simulink model "Kundur_BESS_STA_Nov14_2021a_v2_2021a"  (R2023a)
settings: Solver=VariableStepAuto  StartTime=0.0  StopTime=3  FixedStep=Ts  MaxStep=1e-5  MinStep=1e-20  RelTol=1e-3  EnableMultiTasking=on
PreLoadFcn:
  | Ts=50e-6;
PostLoadFcn:
  | Ts=50e-6;
InitFcn:
  | Ts=50e-6;
values from neighbouring files (symbols this model uses):
  current_K_den = [1 -1.95396088137 0.953960881373]    [param_cntrl_v2.mat]
  current_K_num = [292.549944556 -582.765243791 290.215658722]    [param_cntrl_v2.mat]
  flt_den = [1 -1.99914493247 0.999500180349]    [param_cntrl_v2.mat]
  flt_num = [0.000249925443627 3.12366678454e-08 -0.000249894206959]    [param_cntrl_v2.mat]
  flt_rocof_den = [1 -3.94812243331 5.84544117496 -3.84650440967 0.949185710471]    [param_cntrl_v2.mat]
  flt_rocof_num = [2.65341753303e-09 1.06136701321e-08 1.59205051982e-08 1.06136701321e-08 2.65341753303e-09]    [param_cntrl_v2.mat]
  pll_K_den = [1 -1.95396088137 0.953960881373]    [param_cntrl_v2.mat]
  pll_K_num = [1047.77474974 -2078.89023245 1031.12061217]    [param_cntrl_v2.mat]
  sampling_k = 5e-05    [param_cntrl_v2.mat]
undefined symbols (not defined in the file or in its folder): Ad2, Ad4, Bd2, Bd4, Cd2, Cd4, D1, Delta, flt_rocof_a_den, flt_rocof_a_num, flt_rocof_b_den, flt_rocof_b_num, Gd2, Gd4, Kd2, Kd4, L, R
libraries: spsThreePhaseVIMeasurementLib x15, spsLoadFlowBusLib x12, spsSeriesRLCBranchLib x11, spsThreePhaseSeriesRLCLoadLib x11, spsThreePhaseTransformerTwoWindingsLib x8, spsThreePhaseSeriesRLCBranchLib x8, spsabctoAlphaBetaZeroLib x8, spsGenericPowerSystemStabilizerLib x8, spsPowerPositiveSequenceLib x7, spsThreePhaseParallelRLCLoadLib x6, spsPLL3phLib x6, spsGroundLib x6
(part 2 of 4)

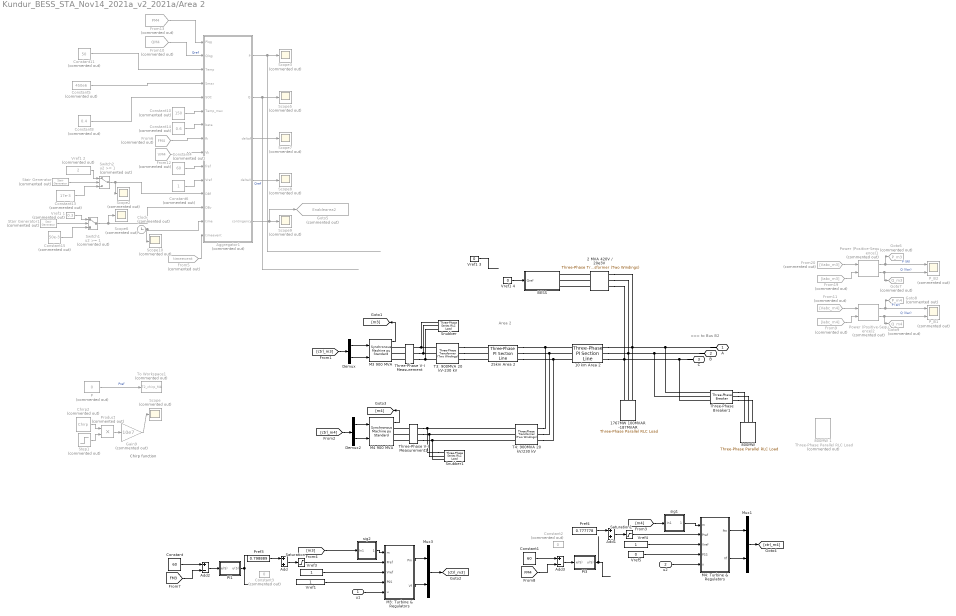
== system Kundur_BESS_STA_Nov14_2021a_v2_2021a/Area 2 ==
  note: ==> to Bus B2
  note: Area 2
  note: Chirp function
  u1 : Inport
  u2 : Inport  Port=2
  10 km Area 2 : spsThreePhasePISectionLineLib/Three-Phase PI Section Line  LConnTagsString=a|b|c  RConnTagsString=A|B|C  Length=10  Frequency=60  Resistances=[0.0001*529 1.61]  Inductances=[0.001*529/(377) 0.0061]  Capacitances=[0.00175/529/(377) 5.2489e-9]
  1767MW 100MVAR -187MVAR : spsThreePhaseParallelRLCLoadLib/Three-Phase Parallel RLC Load  LConnTagsString=A|B|C  Configuration=Y (grounded)  NominalVoltage=230e3  Vabc=[1e3 1e3 1e3]  Vabcp=[1e3 1e3 1e3]  NominalFrequency=60  UnbalancedPower=off  ActivePower=1767e6  InductivePower=0  CapacitivePower=0  Pabc=[10e3 9e3 11e3]  QLabc=[100 90 110]  QCabc=[100 90 110]  Pabcp=[10e3 9e3 11e3]  QLabcp=[100 90 110]  QCabcp=[100 90 110]  Measurements=None  LoadType=constant Z
  2 MVA 420V / 20e3V : spsThreePhaseTransformerTwoWindingsLib/Three-Phase Transformer (Two Windings)  Winding1Connection=Delta (D1)  Winding2Connection=Yg  CoreType=Three single-phase transformers  SetSaturation=off  Hysteresis=off  DataFile='hysteresis'  SetInitialFlux=off  Measurements=None  UNITS=pu  NominalPower=[900e6 , 60 ]  Winding1=[ 20e3 , 0.001 , 0.03 ]  Winding2=[ 420 , 0.001 , 0.03 ]  Rm=500  Lm=500  L0=0.5  Saturation=[ 0,0 ; 0.0024,1.2 ; 1.0,1.52 ]  InitialFluxes=[0.79999 -0.79999 0.7]  BreakLoop=off  DiscreteSolver=Trapezoidal iterative  DataType=off  TransfoNumber=0
  25km Area 2 : spsThreePhasePISectionLineLib/Three-Phase PI Section Line  LConnTagsString=a|b|c  RConnTagsString=A|B|C  Length=25  Frequency=60  Resistances=[0.0001*529 1.61]  Inductances=[0.001*529/(377) 0.0061]  Capacitances=[0.00175/529/(377) 5.2489e-9]
  "800MW " : spsThreePhaseParallelRLCLoadLib/Three-Phase Parallel RLC Load  LConnTagsString=A|B|C  Configuration=Y (grounded)  NominalVoltage=230e3  Vabc=[1e3 1e3 1e3]  Vabcp=[1e3 1e3 1e3]  NominalFrequency=60  UnbalancedPower=off  ActivePower=150e6  InductivePower=0  CapacitivePower=0  Pabc=[10e3 9e3 11e3]  QLabc=[100 90 110]  QCabc=[100 90 110]  Pabcp=[10e3 9e3 11e3]  QLabcp=[100 90 110]  QCabcp=[100 90 110]  Measurements=None  LoadType=constant Z
  800MW 1 : spsThreePhaseParallelRLCLoadLib/Three-Phase Parallel RLC Load  Commented=on  LConnTagsString=A|B|C  Configuration=Y (grounded)  NominalVoltage=230e3  Vabc=[1e3 1e3 1e3]  Vabcp=[1e3 1e3 1e3]  NominalFrequency=60  UnbalancedPower=off  ActivePower=750e6  InductivePower=0  CapacitivePower=0  Pabc=[10e3 9e3 11e3]  QLabc=[100 90 110]  QCabc=[100 90 110]  Pabcp=[10e3 9e3 11e3]  QLabcp=[100 90 110]  QCabcp=[100 90 110]  Measurements=None  LoadType=constant Z
  Add : Sum
  Add1 : Sum
  Add2 : Sum  Inputs=+-
  Add3 : Sum  Inputs=+-
  Aggregator1 : MATLAB Function  Commented=on  TreatAsAtomicUnit=on
  BESS : Subsystem  mask(Off-board charger for EVs){Kp=5, Ki=20, C=3600e-6, Vdc=800, Ts=Ts}
      mask prompts: Kp "Current Controller Kp"; Ki "Current Controller Ki"; C "DC link capacitor [uF]"; Vdc "DC link voltage level [V]"; Ts "Sample period [s]"
      mask help: This model only contains the three phase inverter and current controllers in rotating reference frame (PQ). The DAB converter need to be completed. It only has the inverter to improve the simulation time.
      mask Display: image('parking_lot3.png');
  Chirp2 : dspsrcs4/Chirp  Commented=on  sweep=Logarithmic  mode=Unidirectional  f0=1  f1=1000  t1=10  Tsweep=10  phase=9*pi/8  Ts=Ts  spf=1  datatype=Double  OutputFrames=on
  Clock : Clock  Commented=on
  Constant : Constant  Value=60
  Constant1 : Constant  Value=60
  Constant10 : Constant  Commented=on  Value=150
  Constant11 : Constant  Commented=on  Value=50
  Constant13 : Constant  Commented=on  Value=17e-3
  Constant14 : Constant  Commented=on  Value=0.6
  Constant15 : Constant  Commented=on  Value=50e-3
  Constant2 : Constant  Commented=on  Value=0
  Constant3 : Constant  Commented=on  Value=0
  Constant4 : Constant  Commented=on  Value=60
  Constant5 : Constant  Commented=on  Value=450e6
  Constant6 : Constant  Commented=on
  Constant8 : Constant  Commented=on  Value=0.4
  Demux : Demux  Outputs=[1 1]
  Demux2 : Demux  Outputs=[1 1]
  From10 : From  Commented=on  GotoTag=QM4  TagVisibility=global
  From11 : From  Commented=on  GotoTag=Vabc_m4  TagVisibility=global
      settings: CloseFcn=tagdialog Close
  From12 : From  Commented=on  GotoTag=VM4  TagVisibility=global
  From13 : From  Commented=on  GotoTag=PM4  TagVisibility=global
  From19 : From  Commented=on  GotoTag=Iabc_m3  TagVisibility=global
      settings: CloseFcn=tagdialog Close
  From20 : From  Commented=on  GotoTag=Vabc_m3  TagVisibility=global
      settings: CloseFcn=tagdialog Close
  From5 : From  Commented=on  GotoTag=timeevent  TagVisibility=global
  From6 : From  Commented=on  GotoTag=FM4  TagVisibility=global
  From9 : From  Commented=on  GotoTag=Iabc_m4  TagVisibility=global
      settings: CloseFcn=tagdialog Close
  Gain9 : Gain  Commented=on  Gain=10e7
  Goto5 : Goto  Commented=on  GotoTag=Enablearea2  TagVisibility=global
  Goto6 : Goto  Commented=on  GotoTag=P_m3  TagVisibility=global
  Goto7 : Goto  Commented=on  GotoTag=Q_m3  TagVisibility=global
  Goto8 : Goto  Commented=on  GotoTag=P_m4  TagVisibility=global
  Goto9 : Goto  Commented=on  GotoTag=Q_m4  TagVisibility=global
  M3 900 MVA : spsSynchronousMachinepuStandardLib/Synchronous Machine pu Standard  PresetModel=No  MechanicalLoad=Mechanical power Pm  ShowDetailedParameters=on  RotorType=Round  Units=per unit standard parameters  MeasurementBus=off  NominalParameters="[900E6  20000   60 ]"  Reactances1=[1.8 .3 .25 1.7 .55 .25 .2]  Reactances2=[ 1.305, 0.296, 0.252, 0.474, 0.243, 0.18 ]  dAxisTimeConstants=Open-circuit  qAxisTimeConstants=Open-circuit  TimeConstants1=[]  TimeConstants2=[8 .03 .4 .05]  TimeConstants3=[]  TimeConstants4=[]  TimeConstants5=[ 1.01, 0.053, 0.1 ]  TimeConstants6=[]  TimeConstants7=[]  TimeConstants8=[]  StatorResistance=0.0025  Mechanical="[ 6.175 0  4]"  PolePairs=4  InitialConditions=[0 -56.3243 0.8041 0.8041 0.8041 -22.4087 -142.409 97.5913 1.85092]  SetSaturation=off  Saturation=[0.6404,0.7127,0.8441,0.9214,0.9956,1.082,1.19,1.316,1.457;0.7,0.7698,0.8872,0.9466,0.9969,1.046,1.1,1.151,1.201]  LoadFlowParameters=[1 719000000 0 0 0]  TsPowergui=0  TsBlock=-1  IterativeModel=Trapezoidal non iterative  IterativeDiscreteModel=Trapezoidal non iterative  BusType=PV  Pref=719000000  Qref=0  Qmin=-inf  Qmax=inf  PLF=0  QLF=0
  M3: Turbine & Regulators : Subsystem
  M4 900 MVA : spsSynchronousMachinepuStandardLib/Synchronous Machine pu Standard  PresetModel=No  MechanicalLoad=Mechanical power Pm  ShowDetailedParameters=on  RotorType=Round  Units=per unit standard parameters  MeasurementBus=off  NominalParameters="[900E6  20000   60 ]"  Reactances1=[1.8 .3 .25 1.7 .55 .25 .2]  Reactances2=[ 1.305, 0.296, 0.252, 0.474, 0.243, 0.18 ]  dAxisTimeConstants=Open-circuit  qAxisTimeConstants=Open-circuit  TimeConstants1=[]  TimeConstants2=[8 .03 .4 .05]  TimeConstants3=[]  TimeConstants4=[]  TimeConstants5=[ 1.01, 0.053, 0.1 ]  TimeConstants6=[]  TimeConstants7=[]  TimeConstants8=[]  StatorResistance=0.0025  Mechanical="[ 6.175 0  4]"  PolePairs=4  InitialConditions=[0 -67.7513 0.783185 0.783185 0.783185 -33.268 -153.268 86.732 1.82209]  SetSaturation=off  Saturation=[0.6404,0.7127,0.8441,0.9214,0.9956,1.082,1.19,1.316,1.457;0.7,0.7698,0.8872,0.9466,0.9969,1.046,1.1,1.151,1.201]  LoadFlowParameters=[1 700000000 0 0 0]  TsPowergui=0  TsBlock=-1  IterativeModel=Trapezoidal non iterative  IterativeDiscreteModel=Trapezoidal non iterative  BusType=PV  Pref=700000000  Qref=0  Qmin=-inf  Qmax=inf  PLF=0  QLF=0
  M4: Turbine & Regulators : Subsystem
  Mux1 : Mux  Inputs=2
  Mux3 : Mux  Inputs=2
  P : Constant  Commented=on  Value=0
  PI1 : Subsystem
  PI3 : Subsystem
  P_B1 : Scope  Commented=on  NumInputPorts=2
  P_B2 : Scope  Commented=on  NumInputPorts=2
  Power (Positive-Sequence)1 : spsPowerPositiveSequenceLib/Power (Positive-Sequence)  Commented=on  Freq=60  Vinit=[0, 0]  Iinit=[0, 0]  Ts=Ts
  Power (Positive-Sequence)2 : spsPowerPositiveSequenceLib/Power (Positive-Sequence)  Commented=on  Freq=60  Vinit=[0, 0]  Iinit=[0, 0]  Ts=Ts
  Pref3 : Constant  Value=0.798889
  Pref4 : Constant  Value=0.777778
  Product : Product  Commented=on
  Saturation : Saturate  UpperLimit=1  LowerLimit=0
  Saturation1 : Saturate  UpperLimit=1  LowerLimit=0
  Scope{,2..3,5..10} (9 alike) : Scope  Commented=on
  Snubber : spsThreePhaseSeriesRLCLoadLib/Three-Phase Series RLC Load  LConnTagsString=A|B|C  Configuration=Y (grounded)  NominalVoltage=20000  Vabc=[1e3 1e3 1e3]  Vabcp=[1e3 1e3 1e3]  NominalFrequency=60  UnbalancedPower=off  ActivePower=1e6  InductivePower=0  CapacitivePower=1e7  Pabc=[10e3 9e3 11e3]  QLabc=[100 90 110]  QCabc=[100 90 110]  Pabcp=[10e3 9e3 11e3]  QLabcp=[100 90 110]  QCabcp=[100 90 110]  Measurements=None  LoadType=constant Z
  Snubber1 : spsThreePhaseSeriesRLCLoadLib/Three-Phase Series RLC Load  LConnTagsString=A|B|C  Configuration=Y (grounded)  NominalVoltage=20000  Vabc=[1e3 1e3 1e3]  Vabcp=[1e3 1e3 1e3]  NominalFrequency=60  UnbalancedPower=off  ActivePower=1e6  InductivePower=0  CapacitivePower=1e7  Pabc=[10e3 9e3 11e3]  QLabc=[100 90 110]  QCabc=[100 90 110]  Pabcp=[10e3 9e3 11e3]  QLabcp=[100 90 110]  QCabcp=[100 90 110]  Measurements=None  LoadType=constant Z
  Stair Generator : spsStairGeneratorLib/Stair Generator  Commented=on  t=[0 4]  e=[1 0]  Ts=0
  Stair Generator1 : spsStairGeneratorLib/Stair Generator  Commented=on  t=[0 4]  e=[1 0]  Ts=0
  Step1 : Step  Commented=on  Time=10  SampleTime=0
  Switch1 : Switch  Commented=on  Threshold=1  SaturateOnIntegerOverflow=off
  Switch2 : Switch  Commented=on  Threshold=1  SaturateOnIntegerOverflow=off
  T3: 900MVA 20 kV-230 kV : spsThreePhaseTransformerTwoWindingsLib/Three-Phase Transformer (Two Windings)  Winding1Connection=Delta (D1)  Winding2Connection=Yg  CoreType=Three single-phase transformers  SetSaturation=off  Hysteresis=off  DataFile='hysteresis'  SetInitialFlux=off  Measurements=None  UNITS=pu  NominalPower="[ 900e6   60 ]"  Winding1="[ 20e3  1e-6   0  ]"  Winding2="[ 230e3  1e-6   0.15 ]"  Rm=500  Lm=500  L0=0.5  Saturation="[ 0,0  ;  0.005,1.2  ;  1.0,1.4 ]"  InitialFluxes=[ 0.8 , -0.8 , 0.7 ]  BreakLoop=off  DiscreteSolver=Trapezoidal iterative  DataType=off  TransfoNumber=0
  T4: 900MVA 20 kV/230 kV : spsThreePhaseTransformerTwoWindingsLib/Three-Phase Transformer (Two Windings)  Winding1Connection=Delta (D1)  Winding2Connection=Yg  CoreType=Three single-phase transformers  SetSaturation=off  Hysteresis=off  DataFile='hysteresis'  SetInitialFlux=off  Measurements=None  UNITS=pu  NominalPower=[ 900e6 60 ]  Winding1="[ 20e3 1e-6  0.0]"  Winding2=[ 230e3 1e-6 0.15]  Rm=500  Lm=500  L0=0.5  Saturation="[ 0,0  ;  0.005,1.2  ;  1.0,1.4 ]"  InitialFluxes=[ 0.8 , -0.8 , 0.7 ]  BreakLoop=off  DiscreteSolver=Trapezoidal iterative  DataType=off  TransfoNumber=0
  Three-Phase V-I Measurement : spsThreePhaseVIMeasurementLib/Three-Phase V-I Measurement  VoltageMeasurement=phase-to-ground  SetLabelV=on  LabelV=Vabc_m3  Vpu=off  VpuLL=off  CurrentMeasurement=yes  SetLabelI=on  LabelI=Iabc_m3  Ipu=off  Pbase=100e6  Vbase=500e3  OutputType=Complex  PhasorSimulation=off  PSBequivalent=0
  Three-Phase V-I Measurement1 : spsThreePhaseVIMeasurementLib/Three-Phase V-I Measurement  VoltageMeasurement=phase-to-ground  SetLabelV=on  LabelV=Vabc_m4  Vpu=off  VpuLL=off  CurrentMeasurement=yes  SetLabelI=on  LabelI=Iabc_m4  Ipu=off  Pbase=100e6  Vbase=500e3  OutputType=Complex  PhasorSimulation=off  PSBequivalent=0
  Three-Phase Breaker1 : spsThreePhaseBreakerLib/Three-Phase Breaker  InitialState=open  SwitchA=on  SwitchB=on  SwitchC=on  SwitchTimes=[1.5]  External=off  BreakerResistance=0.01  SnubberResistance=1e6  SnubberCapacitance=inf  Measurements=None
  To Workspace1 : ToWorkspace  Commented=on  VariableName=T2_chirp_M4  SampleTime=Ts
      settings: Save2DSignal=2-D array (concatenate along first dimension)
  Vref1 : Constant
  Vref1 1 : Constant  Commented=on  Value=0.3
  Vref1 2 : Constant  Commented=on  Value=2
  Vref1 3 : Constant  Value=0
  Vref1 4 : Constant  Value=0
  Vref3 : Constant
  Vref4 : Constant
  Vref5 : Constant  Value=0
  sig1 : Subsystem
  sig2 : Subsystem
  A : PMIOPort  Side=Left
  B : PMIOPort  Port=2  Side=Left
  C : PMIOPort  Port=3  Side=Left
  wires:
  Vref3/1 -> M3: Turbine & Regulators/3(Vref)
  Vref4/1 -> M4: Turbine & Regulators/3(Vref)
  Vref5/1 -> M4: Turbine & Regulators/4(PSS)
  M3 900 MVA/1 -> [m3]
  M4 900 MVA/1 -> [m4]
  [ctrl_m3] -> Demux/1
  Demux/1 -> M3 900 MVA/1
  Demux/2 -> M3 900 MVA/2
  [ctrl_m4] -> Demux2/1
  Demux2/2 -> M4 900 MVA/2
  Demux2/1 -> M4 900 MVA/1
  Mux3/1 -> [ctrl_m3]
  M3: Turbine & Regulators/2(Vf) -> Mux3/2
  M3: Turbine & Regulators/1(Pm) -> Mux3/1
  sig2/1(Out1) -> M3: Turbine & Regulators/1(m)
  Mux1/1 -> [ctrl_m4]
  M4: Turbine & Regulators/1(Pm) -> Mux1/1
  M4: Turbine & Regulators/2(Vf) -> Mux1/2
  sig1/1(Out1) -> M4: Turbine & Regulators/1(m)
  [m4] -> sig1/1(In1)
  [m3] -> sig2/1(In1)
  Vref1/1 -> M3: Turbine & Regulators/4(PSS)
  u1/1 -> M3: Turbine & Regulators/5(u)
  u2/1 -> M4: Turbine & Regulators/5(u)
  Saturation/1 -> M3: Turbine & Regulators/2(Pref)
  Product/1 -> Gain9/1
  Chirp2/1 -> Product/1
  Step1/1 -> Product/2
  Gain9/1 -> Scope/1
  P/1 -> To Workspace1/1  "Pref"
  Aggregator1/1(P) -> Scope3/1
  Aggregator1/2(Q) -> Scope5/1  "Qref"
  Add/1 -> Saturation/1
  Pref3/1 -> Add/1
  Pref4/1 -> Add1/1
  Add1/1 -> Saturation1/1
  Saturation1/1 -> M4: Turbine & Regulators/2(Pref)
  [FM3] -> Add2/2
  PI1/1(u(S)) -> ?
  Constant/1 -> Add2/1
  Add2/1 -> PI1/1(e(S))
  Add3/1 -> PI3/1(e(S))
  Constant1/1 -> Add3/1
  PI3/1(u(S)) -> ?
  [FM4] -> Add3/2
  From20/1 -> Power (Positive-Sequence)1/1
  Power (Positive-Sequence)1/2 -> Goto7/1, P_B2/2  "Q (Var)"
  From19/1 -> Power (Positive-Sequence)1/2
  From11/1 -> Power (Positive-Sequence)2/1
  Power (Positive-Sequence)2/2 -> Goto9/1, P_B1/2  "Q (Var)"
  Power (Positive-Sequence)1/1 -> Goto6/1, P_B2/1  "P (W)"
  From9/1 -> Power (Positive-Sequence)2/2
  Power (Positive-Sequence)2/1 -> Goto8/1, P_B1/1  "P (W)"
  Aggregator1/3(deltaf) -> Scope7/1
  Switch1/1 -> Scope6/1, Aggregator1/13(DBv)
  Constant8/1 -> Aggregator1/5(SOC)
  From12/1 -> Aggregator1/9(Vk)
  Constant4/1 -> Aggregator1/10(fref)
  From6/1 -> Aggregator1/8(fk)
  Clock/1 -> Aggregator1/14(time), Scope10/1
  From10/1 -> Aggregator1/2(Qlqg)  "Qref"
  Constant14/1 -> Aggregator1/7(beta)
  Constant5/1 -> Aggregator1/4(Smax)
  From13/1 -> Aggregator1/1(Plqg)
  Constant11/1 -> Aggregator1/3(Temp)
  Constant10/1 -> Aggregator1/6(Temp_max)
  Constant6/1 -> Aggregator1/11(Vref)
  Aggregator1/5(contingency) -> Goto5/1, Scope9/1
  Aggregator1/4(deltaV) -> Scope8/1
  From5/1 -> Aggregator1/15(timeevent)
  Vref1 2/1 -> Switch2/1
  Constant13/1 -> Switch2/3
  Stair Generator/1 -> Switch2/2
  Switch2/1 -> Scope2/1, Aggregator1/12(DBf)
  Stair Generator1/1 -> Switch1/2
  Vref1 1/1 -> Switch1/1
  Constant15/1 -> Switch1/3
  Vref1 3/1 -> ?
  Vref1 4/1 -> BESS/1(Qref)
  connections:
  T3: 900MVA 20 kV-230 kV/LConn3 -- Three-Phase V-I Measurement/RConn3 -- Snubber/LConn3
  T3: 900MVA 20 kV-230 kV/LConn2 -- Three-Phase V-I Measurement/RConn2 -- Snubber/LConn2
  Snubber/LConn1 -- T3: 900MVA 20 kV-230 kV/LConn1 -- Three-Phase V-I Measurement/RConn1
  T3: 900MVA 20 kV-230 kV/RConn3 -- 25km Area 2/LConn3
  Snubber1/LConn3 -- T4: 900MVA 20 kV/230 kV/LConn3 -- Three-Phase V-I Measurement1/RConn3
  T4: 900MVA 20 kV/230 kV/LConn2 -- Three-Phase V-I Measurement1/RConn2 -- Snubber1/LConn2
  Snubber1/LConn1 -- T4: 900MVA 20 kV/230 kV/LConn1 -- Three-Phase V-I Measurement1/RConn1
  T3: 900MVA 20 kV-230 kV/RConn2 -- 25km Area 2/LConn2
  T3: 900MVA 20 kV-230 kV/RConn1 -- 25km Area 2/LConn1
  10 km Area 2/RConn2 -- Three-Phase Breaker1/LConn2 -- B/RConn1 -- 2 MVA 420V / 20e3V/LConn2 -- 1767MW 100MVAR -187MVAR/LConn2
  10 km Area 2/RConn1 -- Three-Phase Breaker1/LConn1 -- A/RConn1 -- 2 MVA 420V / 20e3V/LConn1 -- 1767MW 100MVAR -187MVAR/LConn3
  25km Area 2/RConn2 -- 10 km Area 2/LConn2 -- T4: 900MVA 20 kV/230 kV/RConn2
  25km Area 2/RConn1 -- 10 km Area 2/LConn1 -- T4: 900MVA 20 kV/230 kV/RConn1
  25km Area 2/RConn3 -- 10 km Area 2/LConn3 -- T4: 900MVA 20 kV/230 kV/RConn3
  2 MVA 420V / 20e3V/RConn3 -- BESS/RConn3
  2 MVA 420V / 20e3V/RConn2 -- BESS/RConn2
  2 MVA 420V / 20e3V/RConn1 -- BESS/RConn1
  Three-Phase V-I Measurement/LConn1 -- M3 900 MVA/RConn1
  Three-Phase V-I Measurement/LConn2 -- M3 900 MVA/RConn2
  Three-Phase V-I Measurement/LConn3 -- M3 900 MVA/RConn3
  Three-Phase V-I Measurement1/LConn1 -- M4 900 MVA/RConn1
  Three-Phase V-I Measurement1/LConn2 -- M4 900 MVA/RConn2
  Three-Phase V-I Measurement1/LConn3 -- M4 900 MVA/RConn3
  Three-Phase Breaker1/RConn3 -- "800MW "/LConn3
  Three-Phase Breaker1/RConn1 -- "800MW "/LConn1
  Three-Phase Breaker1/RConn2 -- "800MW "/LConn2
  10 km Area 2/RConn3 -- Three-Phase Breaker1/LConn3 -- C/RConn1 -- 2 MVA 420V / 20e3V/LConn3 -- 1767MW 100MVAR -187MVAR/LConn1

== system Kundur_BESS_STA_Nov14_2021a_v2_2021a/LQG2 ==
  y(t) : Inport
  Enable : EnablePort
  Gain10 : Gain  Gain=-Gd2  Multiplication=Matrix(K*u)
  Gain11 : Gain  Gain=Bd2  Multiplication=Matrix(K*u)
  Gain12 : Gain  Gain=-Kd2'  Multiplication=Matrix(K*u)
  Gain13 : Gain  Gain=Cd2  Multiplication=Matrix(K*u)
  Gain14 : Gain  Gain=Ad2  Multiplication=Matrix(K*u)
  Sum5 : Sum  Inputs=|++
  Sum6 : Sum  Inputs=+++
  Unit Delay : UnitDelay  InitialCondition=zeros(size(Ad2(1,:)))  SampleTime=Ts  HasFrameUpgradeWarning=on
  u(t) : Outport  VectorParamsAs1DForOutWhenUnconnected=off
  wires:
  Sum5/1 -> Gain10/1
  Unit Delay/1 -> Gain13/1, Gain14/1, Gain12/1
  Gain14/1 -> Sum6/3
  Gain13/1 -> Sum5/2
  y(t)/1 -> Sum5/1
  Gain10/1 -> Sum6/2
  Gain11/1 -> Sum6/1
  Sum6/1 -> Unit Delay/1
  Gain12/1 -> u(t)/1, Gain11/1

== system Kundur_BESS_STA_Nov14_2021a_v2_2021a/LQG4 ==
  y(t) : Inport
  Enable : EnablePort
  Gain10 : Gain  Gain=-Gd4  Multiplication=Matrix(K*u)
  Gain11 : Gain  Gain=Bd4  Multiplication=Matrix(K*u)
  Gain12 : Gain  Gain=-Kd4'  Multiplication=Matrix(K*u)
  Gain13 : Gain  Gain=Cd4  Multiplication=Matrix(K*u)
  Gain14 : Gain  Gain=Ad4  Multiplication=Matrix(K*u)
  Sum5 : Sum  Inputs=|++
  Sum6 : Sum  Inputs=+++
  Unit Delay : UnitDelay  InitialCondition=zeros(size(Ad2(1,:)))  SampleTime=Ts  HasFrameUpgradeWarning=on
  u(t) : Outport  VectorParamsAs1DForOutWhenUnconnected=off
  wires:
  Sum5/1 -> Gain10/1
  Unit Delay/1 -> Gain13/1, Gain14/1, Gain12/1
  Gain14/1 -> Sum6/3
  Gain13/1 -> Sum5/2
  y(t)/1 -> Sum5/1
  Gain10/1 -> Sum6/2
  Gain11/1 -> Sum6/1
  Sum6/1 -> Unit Delay/1
  Gain12/1 -> u(t)/1, Gain11/1

== system Kundur_BESS_STA_Nov14_2021a_v2_2021a/Model Initialization1 ==

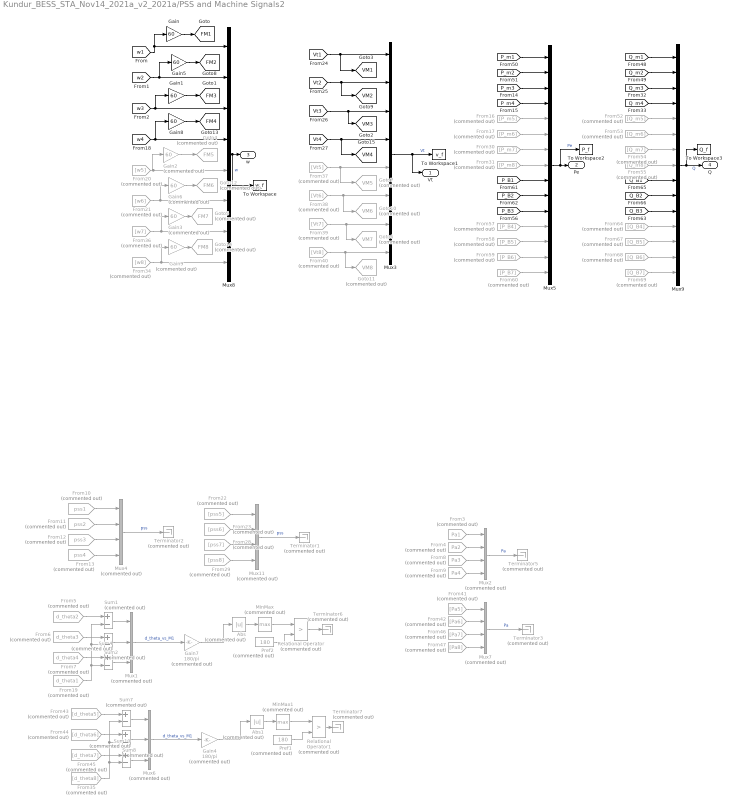
== system Kundur_BESS_STA_Nov14_2021a_v2_2021a/PSS and Machine Signals2 ==
  Abs : Abs  Commented=on
  Abs1 : Abs  Commented=on
  From10 : From  Commented=on  GotoTag=pss1  TagVisibility=global
      settings: CloseFcn=tagdialog Close
  From11 : From  Commented=on  GotoTag=pss2  TagVisibility=global
      settings: CloseFcn=tagdialog Close
  From12 : From  Commented=on  GotoTag=pss3  TagVisibility=global
      settings: CloseFcn=tagdialog Close
  From13 : From  Commented=on  GotoTag=pss4  TagVisibility=global
      settings: CloseFcn=tagdialog Close
  From16 : From  Commented=on  GotoTag=P_m5
  From17 : From  Commented=on  GotoTag=P_m6
  From19 : From  Commented=on  GotoTag=d_theta1  TagVisibility=global
      settings: CloseFcn=tagdialog Close
  From20 : From  Commented=on  GotoTag=w5
      settings: CloseFcn=tagdialog Close
  From21 : From  Commented=on  GotoTag=w6
      settings: CloseFcn=tagdialog Close
  From22 : From  Commented=on  GotoTag=pss5  TagVisibility=global
      settings: CloseFcn=tagdialog Close
  From23 : From  Commented=on  GotoTag=pss6  TagVisibility=global
      settings: CloseFcn=tagdialog Close
  From28 : From  Commented=on  GotoTag=pss7  TagVisibility=global
      settings: CloseFcn=tagdialog Close
  From29 : From  Commented=on  GotoTag=pss8  TagVisibility=global
      settings: CloseFcn=tagdialog Close
  From3 : From  Commented=on  GotoTag=Pa1  TagVisibility=global
      settings: CloseFcn=tagdialog Close
  From30 : From  Commented=on  GotoTag=P_m7
  From31 : From  Commented=on  GotoTag=P_m8
  From34 : From  Commented=on  GotoTag=w8
      settings: CloseFcn=tagdialog Close
  From35 : From  Commented=on  GotoTag=d_theta8  TagVisibility=global
      settings: CloseFcn=tagdialog Close
  From36 : From  Commented=on  GotoTag=w7
      settings: CloseFcn=tagdialog Close
  From37 : From  Commented=on  GotoTag=Vt5
      settings: CloseFcn=tagdialog Close
  From38 : From  Commented=on  GotoTag=Vt6
      settings: CloseFcn=tagdialog Close
  From39 : From  Commented=on  GotoTag=Vt7
      settings: CloseFcn=tagdialog Close
  From4 : From  Commented=on  GotoTag=Pa2  TagVisibility=global
      settings: CloseFcn=tagdialog Close
  From40 : From  Commented=on  GotoTag=Vt8
      settings: CloseFcn=tagdialog Close
  From41 : From  Commented=on  GotoTag=Pa5  TagVisibility=global
      settings: CloseFcn=tagdialog Close
  From42 : From  Commented=on  GotoTag=Pa6  TagVisibility=global
      settings: CloseFcn=tagdialog Close
  From43 : From  Commented=on  GotoTag=d_theta5  TagVisibility=global
      settings: CloseFcn=tagdialog Close
  From44 : From  Commented=on  GotoTag=d_theta6  TagVisibility=global
      settings: CloseFcn=tagdialog Close
  From45 : From  Commented=on  GotoTag=d_theta7  TagVisibility=global
      settings: CloseFcn=tagdialog Close
  From46 : From  Commented=on  GotoTag=Pa7  TagVisibility=global
      settings: CloseFcn=tagdialog Close
  From47 : From  Commented=on  GotoTag=Pa8  TagVisibility=global
      settings: CloseFcn=tagdialog Close
  From5 : From  Commented=on  GotoTag=d_theta2  TagVisibility=global
      settings: CloseFcn=tagdialog Close
  From52 : From  Commented=on  GotoTag=Q_m5
  From53 : From  Commented=on  GotoTag=Q_m6
  From54 : From  Commented=on  GotoTag=Q_m7
  From55 : From  Commented=on  GotoTag=Q_m8
  From57 : From  Commented=on  GotoTag=P_B4
  From58 : From  Commented=on  GotoTag=P_B5
  From59 : From  Commented=on  GotoTag=P_B6
  From6 : From  Commented=on  GotoTag=d_theta3  TagVisibility=global
      settings: CloseFcn=tagdialog Close
  From60 : From  Commented=on  GotoTag=P_B7
  From64 : From  Commented=on  GotoTag=Q_B4
  From67 : From  Commented=on  GotoTag=Q_B5
  From68 : From  Commented=on  GotoTag=Q_B6
  From69 : From  Commented=on  GotoTag=Q_B7
  From7 : From  Commented=on  GotoTag=d_theta4  TagVisibility=global
      settings: CloseFcn=tagdialog Close
  From8 : From  Commented=on  GotoTag=Pa3  TagVisibility=global
      settings: CloseFcn=tagdialog Close
  From9 : From  Commented=on  GotoTag=Pa4  TagVisibility=global
      settings: CloseFcn=tagdialog Close
  Gain{,1,5,8} (4 alike) : Gain  Gain=60
  Gain{2..3,6,9} (4 alike) : Gain  Commented=on  Gain=60
  Gain4 : Gain  Commented=on  Gain=180/pi
  Gain7 : Gain  Commented=on  Gain=180/pi
  Goto10 : Goto  Commented=on  GotoTag=VM6  TagVisibility=global
  Goto11 : Goto  Commented=on  GotoTag=VM8  TagVisibility=global
  Goto12 : Goto  Commented=on  GotoTag=FM6  TagVisibility=global
  Goto14 : Goto  Commented=on  GotoTag=FM8  TagVisibility=global
  Goto4 : Goto  Commented=on  GotoTag=FM5  TagVisibility=global
  Goto5 : Goto  Commented=on  GotoTag=FM7  TagVisibility=global
  Goto6 : Goto  Commented=on  GotoTag=VM7  TagVisibility=global
  Goto7 : Goto  Commented=on  GotoTag=VM5  TagVisibility=global
  MinMax : MinMax  Commented=on  Function=max  InputSameDT=on  SaturateOnIntegerOverflow=on
  MinMax1 : MinMax  Commented=on  Function=max  InputSameDT=on  SaturateOnIntegerOverflow=on
  Mux1 : Mux  Commented=on  Inputs=3
  Mux{2,4,7,11} (4 alike) : Mux  Commented=on
  Mux3 : Mux  Inputs=8
  Mux5 : Mux  Inputs=15
  Mux6 : Mux  Commented=on  Inputs=3
  Mux8 : Mux  Inputs=8
  Mux9 : Mux  Inputs=15
  Pref1 : Constant  Commented=on  Value=180
  Pref2 : Constant  Commented=on  Value=180
  Relational Operator : RelationalOperator  Commented=on  Operator=>
  Relational Operator1 : RelationalOperator  Commented=on  Operator=>
  Sum{1..2,4,7..8,10} (6 alike) : Sum  Commented=on  Inputs=+-  InputSameDT=on  SaturateOnIntegerOverflow=on  OutDataTypeStr=Inherit: Same as first input
  Terminator{1..3,5..7} (6 alike) : Terminator  Commented=on
  To Workspace : ToWorkspace  VariableName=w_f  SampleTime=Ts
      settings: Save2DSignal=2-D array (concatenate along first dimension)
  To Workspace1 : ToWorkspace  VariableName=v_f  SampleTime=Ts
      settings: Save2DSignal=2-D array (concatenate along first dimension)
  To Workspace2 : ToWorkspace  VariableName=P_f  SampleTime=Ts
      settings: Save2DSignal=2-D array (concatenate along first dimension)
  To Workspace3 : ToWorkspace  VariableName=Q_f  SampleTime=Ts
      settings: Save2DSignal=2-D array (concatenate along first dimension)
  Vt : Outport  VectorParamsAs1DForOutWhenUnconnected=off
  "Pe " : Outport  Port=2  VectorParamsAs1DForOutWhenUnconnected=off
  w : Outport  Port=3  VectorParamsAs1DForOutWhenUnconnected=off
  Q : Outport  Port=4  VectorParamsAs1DForOutWhenUnconnected=off
  tag scope: FM1=global, FM2=global, FM3=global, FM4=global, VM1=global, VM2=global, VM3=global, VM4=global
  wires:
  From3/1 -> Mux2/1
  Mux4/1 -> Terminator2/1  "pss"
  From10/1 -> Mux4/1
  From11/1 -> Mux4/2
  From13/1 -> Mux4/4
  From12/1 -> Mux4/3
  Mux8/1 -> To Workspace/1, w/1  "w"
  Relational Operator/1 -> Terminator6/1
  Mux2/1 -> Terminator5/1  "Pa"
  From4/1 -> Mux2/2
  From8/1 -> Mux2/3
  From9/1 -> Mux2/4
  [Vt1] -> [VM1], Mux3/1
  [Vt2] -> [VM2], Mux3/2
  [Vt3] -> Mux3/3, [VM3]
  [Vt4] -> [VM4], Mux3/4
  Mux3/1 -> To Workspace1/1, Vt/1  "Vt"
  [P_m1] -> Mux5/1
  [P_m2] -> Mux5/2
  [P_m3] -> Mux5/3
  [P_m4] -> Mux5/4
  Mux5/1 -> To Workspace2/1, "Pe "/1  "Pe"
  [w1] -> Gain/1, Mux8/1
  Mux1/1 -> Gain7/1  "d_theta_vs_M1"
  Abs/1 -> MinMax/1
  Pref2/1 -> Relational Operator/2
  MinMax/1 -> Relational Operator/1
  From5/1 -> Sum1/1
  Sum1/1 -> Mux1/1
  From6/1 -> Sum2/1
  From7/1 -> Sum4/1
  From19/1 -> Sum4/2, Sum2/2, Sum1/2
  Sum2/1 -> Mux1/2
  Sum4/1 -> Mux1/3
  Gain7/1 -> Abs/1
  Gain/1 -> [FM1]
  [w3] -> Gain1/1, Mux8/3
  Gain1/1 -> [FM3]
  Gain4/1 -> Abs1/1
  From29/1 -> Mux11/4
  From35/1 -> Sum10/2, Sum8/2, Sum7/2
  From36/1 -> Gain3/1, Mux8/7
  Gain2/1 -> Goto4/1
  From22/1 -> Mux11/1
  Sum10/1 -> Mux6/3
  Sum8/1 -> Mux6/2
  From44/1 -> Sum8/1
  Pref1/1 -> Relational Operator1/2
  MinMax1/1 -> Relational Operator1/1
  From16/1 -> Mux5/5
  Gain3/1 -> Goto5/1
  From17/1 -> Mux5/6
  From23/1 -> Mux11/2
  From43/1 -> Sum7/1
  Mux6/1 -> Gain4/1  "d_theta_vs_M1"
  Abs1/1 -> MinMax1/1
  From31/1 -> Mux5/8
  From28/1 -> Mux11/3
  From20/1 -> Gain2/1, Mux8/5
  Sum7/1 -> Mux6/1
  From30/1 -> Mux5/7
  From47/1 -> Mux7/4
  From46/1 -> Mux7/3
  From45/1 -> Sum10/1
  From41/1 -> Mux7/1
  From42/1 -> Mux7/2
  Mux11/1 -> Terminator1/1  "pss"
  Mux7/1 -> Terminator3/1  "Pa"
  From40/1 -> Goto11/1, Mux3/8
  From38/1 -> Goto10/1, Mux3/6
  From39/1 -> Mux3/7, Goto6/1
  From37/1 -> Goto7/1, Mux3/5
  Gain5/1 -> [FM2]
  [w2] -> Gain5/1, Mux8/2
  From53/1 -> Mux9/6
  [Q_m1] -> Mux9/1
  From54/1 -> Mux9/7
  Mux9/1 -> To Workspace3/1, Q/1  "Q"
  From52/1 -> Mux9/5
  [Q_m3] -> Mux9/3
  [Q_m2] -> Mux9/2
  [Q_m4] -> Mux9/4
  From55/1 -> Mux9/8
  [P_B2] -> Mux5/10
  From60/1 -> Mux5/15
  [P_B1] -> Mux5/9
  From59/1 -> Mux5/14
  [P_B3] -> Mux5/11
  From57/1 -> Mux5/12
  From58/1 -> Mux5/13
  From67/1 -> Mux9/13
  [Q_B3] -> Mux9/11
  [Q_B1] -> Mux9/9
  From64/1 -> Mux9/12
  [Q_B2] -> Mux9/10
  From69/1 -> Mux9/15
  From68/1 -> Mux9/14
  From21/1 -> Gain6/1, Mux8/6
  Gain6/1 -> Goto12/1
  Gain8/1 -> [FM4]
  [w4] -> Gain8/1, Mux8/4
  Gain9/1 -> Goto14/1
  From34/1 -> Gain9/1, Mux8/8
  Relational Operator1/1 -> Terminator7/1

== system Kundur_BESS_STA_Nov14_2021a_v2_2021a/Subsystem3 ==
  Measurements : Inport
  Add : Sum  Commented=on  Inputs=-+
  Add1 : Sum  Commented=on  Inputs=+-
  Add2 : Sum  Inputs=+-
  Constant : Constant  Commented=on  Value=2
  Constant1 : Constant  Commented=on  Value=2
  Constant3 : Constant
  Demux : Demux  Commented=on
  Divide : Product  Commented=on  Inputs=*/
  Divide1 : Product  Commented=on  Inputs=*/
  Gain : Gain  Commented=on  Gain=-1
  Gain1 : Gain  Commented=on  Gain=150
  Gain3 : Gain  Gain=-1
  Gain4 : Gain  Gain=100
  Gain5 : Gain  Gain=0.00001
  Memory1 : Memory  InitialCondition=[0 0 0 0 0 0 0 0]
  Mux : Mux  Commented=on
  Sum : Sum  Commented=on  Inputs=|++
  Sum2 : Sum  Commented=on  Inputs=|++
  Sum3 : Sum  Commented=on  Inputs=|++
  Sum4 : Sum  Inputs=|++
  Sum5 : Sum  Inputs=|++
  Control : Outport  VectorParamsAs1DForOutWhenUnconnected=off
  wires:
  Add/1 -> Mux/2, Mux/1
  Divide1/1 -> Add1/2, Add/2
  Divide/1 -> Add/1, Add1/1
  Sum3/1 -> Divide1/1
  Constant1/1 -> Divide1/2
  Constant/1 -> Divide/2
  Sum2/1 -> Divide/1
  Demux/4 -> Sum3/2
  Demux/3 -> Sum3/1
  Demux/2 -> Sum2/2
  Demux/1 -> Sum2/1
  Mux/1 -> Gain/1
  Gain/1 -> Gain1/1
  Gain1/1 -> Sum/1
  Memory1/1 -> Sum5/2
  Sum5/1 -> Sum4/2, Memory1/1
  Gain4/1 -> Sum4/1
  Gain5/1 -> Sum5/1
  Add2/1 -> Gain3/1
  Gain3/1 -> Gain5/1, Gain4/1
  Measurements/1 -> Add2/2, Demux/1
  Constant3/1 -> Add2/1
  Add1/1 -> Mux/4, Mux/3
  Sum4/1 -> Control/1

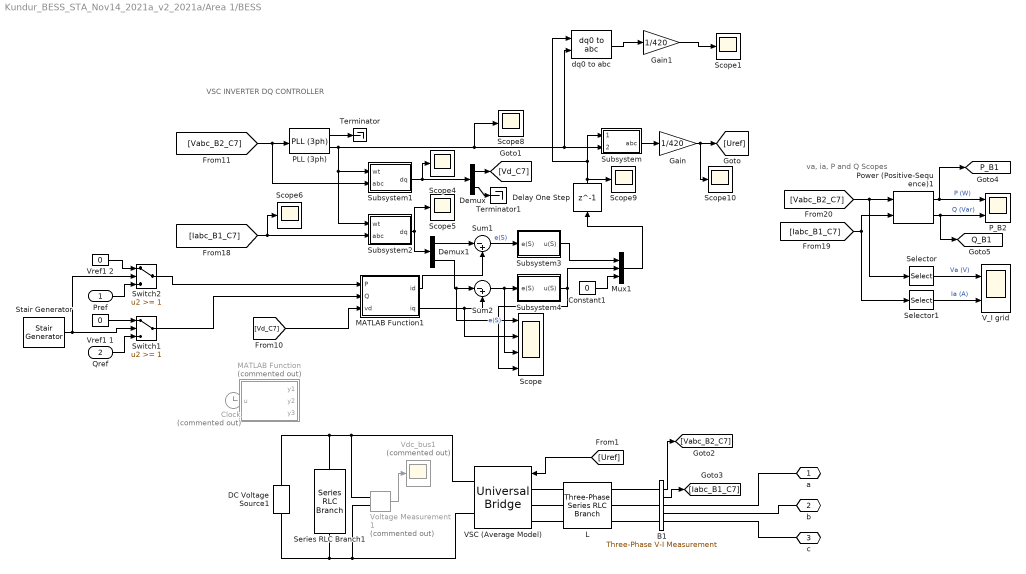
== system Kundur_BESS_STA_Nov14_2021a_v2_2021a/Area 1/BESS ==
  note: VSC INVERTER DQ CONTROLLER
  note: va, ia, P and Q Scopes
  Pref : Inport
  Qref : Inport  Port=2
  B1 : spsThreePhaseVIMeasurementLib/Three-Phase V-I Measurement  VoltageMeasurement=phase-to-ground  SetLabelV=off  LabelV=Vabc_B1  Vpu=off  VpuLL=off  CurrentMeasurement=yes  SetLabelI=off  LabelI=Iabc_B1_C7  Ipu=off  Pbase=100e6  Vbase=500e3  OutputType=Magnitude  PhasorSimulation=off  PSBequivalent=0
  Clock : Clock  Commented=on
  Constant1 : Constant  Value=0
  DC Voltage Source1 : spsDCVoltageSourceLib/DC Voltage Source  Amplitude=Vdc  Measurements=None
  Delay One Step : Delay  DelayLength=1
  Demux : Demux  Outputs=2
  Demux1 : Demux  Outputs=2
  Gain : Gain  Gain=1/420
  Gain1 : Gain  Gain=1/420
  L : spsThreePhaseSeriesRLCBranchLib/Three-Phase Series RLC Branch  LConnTagsString=A|B|C  RConnTagsString=A|B|C  BranchType=RL  Resistance=500e-6*377/50/2  Inductance=1200e-6/2  Capacitance=inf  Measurements=None
  MATLAB Function : MATLAB Function  Commented=on  TreatAsAtomicUnit=on
  MATLAB Function1 : MATLAB Function  TreatAsAtomicUnit=on
  Mux1 : Mux  Inputs=3
  PLL (3ph) : spsPLL3phLib/PLL (3ph)  Fmin=58  Par_Init="[-0.57  60]"  ParK=[180, 3200, 1]  TcD=1e-4  MaxRateChangeFreq=12  FilterCutOffFreq=25  Ts=Ts  AGC=on
  P_B2 : Scope  NumInputPorts=2
  Power (Positive-Sequence)1 : spsPowerPositiveSequenceLib/Power (Positive-Sequence)  Freq=60  Vinit=[0, 0]  Iinit=[0, 0]  Ts=Ts
  Scope : Scope  NumInputPorts=4
  Scope{1,4..6,8..10} (7 alike) : Scope
  Selector : Selector  InputPortWidth=3  IndexOptions=Index vector (dialog)  Indices=[1]  OutputSizes=1
  Selector1 : Selector  InputPortWidth=3  IndexOptions=Index vector (dialog)  Indices=[1]  OutputSizes=1
  Series RLC Branch1 : spsSeriesRLCBranchLib/Series RLC Branch  LConnTagsString=__new0  RConnTagsString=__new0  BranchType=RC  Resistance=1e-7  Inductance=1e-3  SetiL0=off  InitialCurrent=0  Capacitance=C  Setx0=off  InitialVoltage=400  Measurements=None
  Stair Generator : spsStairGeneratorLib/Stair Generator  t=[0 0.03]  e=[1 0]  Ts=0
  Subsystem : Subsystem
  Subsystem1 : Subsystem
  Subsystem2 : Subsystem
  Subsystem3 : Subsystem
  Subsystem4 : Subsystem
  Sum1 : Sum  Inputs=|-+
  Sum2 : Sum  Inputs=|-+
  Switch1 : Switch  Threshold=1  SaturateOnIntegerOverflow=off
  Switch2 : Switch  Threshold=1  SaturateOnIntegerOverflow=off
  Terminator : Terminator
  Terminator1 : Terminator
  VSC (Average Model) : spsUniversalBridgeLib/Universal Bridge  Arms=3  SnubberResistance=1e5  SnubberCapacitance=inf  Device=Average-model based VSC  Ron=1e-3  Lon=0  ForwardVoltages="[  0  0  ]"  ForwardVoltage=0  GTOparameters=[ 10e-6 , 20e-6 ]  IGBTparameters=[ 1e-6 , 2e-6 ]  Measurements=None  Measurements_2=None  converterType=Rectifier
  V_I grid : Scope  NumInputPorts=2
  Vdc_bus1 : Scope  Commented=on
  Voltage Measurement1 : spsVoltageMeasurementLib/Voltage Measurement  Commented=on  PhasorSimulation=off  OutputType=Complex  PSBequivalent=0
  Vref1 1 : Constant  Value=0
  Vref1 2 : Constant  Value=0
  dq0 to abc : spsdq0toabcLib/dq0 to abc  Alignment=90 degrees behind phase A axis
  a : PMIOPort  Side=Right
  b : PMIOPort  Port=2  Side=Right
  c : PMIOPort  Port=3  Side=Right
  tag scope: P_B1=global, Q_B1=global
  wires:
  Sum2/1 -> Scope/3, Subsystem4/1(e(S))  "e(S)"
  PLL (3ph)/2 -> Subsystem2/1(wt), Subsystem1/1(wt), Scope8/1, dq0 to abc/2, Subsystem/2(wt1)
  Voltage Measurement1/1 -> Vdc_bus1/1
  Mux1/1 -> Delay One Step/1
  Selector/1 -> V_I grid/1  "Va (V)"
  Delay One Step/1 -> Scope9/1, dq0 to abc/1, Subsystem/1(dq0)
  MATLAB Function1/1(id) -> Sum1/2
  Sum1/1 -> Subsystem3/1(e(S))  "e(S)"
  Subsystem4/1(u(S)) -> Mux1/2, Scope/4
  Power (Positive-Sequence)1/2 -> [Q_B1], P_B2/2  "Q (Var)"
  Demux/1 -> [Vd_C7]
  [Iabc_B1_C7] -> Scope6/1, Subsystem2/2(abc)
  Subsystem/1(abc) -> Gain/1
  [Vabc_B2_C7] -> Selector/1, Power (Positive-Sequence)1/1
  Subsystem3/1(u(S)) -> Mux1/1
  Gain/1 -> Scope10/1, [Uref]
  [Vabc_B2_C7] -> Subsystem1/2(abc), PLL (3ph)/1
  Selector1/1 -> V_I grid/2  "Ia (A)"
  Demux1/1 -> Sum1/1
  [Uref] -> VSC (Average Model)/1
  Demux/2 -> Terminator1/1
  [Iabc_B1_C7] -> Power (Positive-Sequence)1/2, Selector1/1
  Constant1/1 -> Mux1/3
  Subsystem1/1(dq) -> Demux/1, Scope4/1
  Demux1/2 -> Scope/1, Sum2/1
  Power (Positive-Sequence)1/1 -> [P_B1], P_B2/1  "P (W)"
  MATLAB Function1/2(iq) -> Scope/2, Sum2/2
  [Vd_C7] -> MATLAB Function1/3(vd)
  PLL (3ph)/1 -> Terminator/1
  Subsystem2/1(dq) -> Demux1/1, Scope5/1
  B1/1 -> [Vabc_B2_C7]
  B1/2 -> [Iabc_B1_C7]
  Clock/1 -> MATLAB Function/1(u)
  Qref/1 -> Switch1/3
  Vref1 1/1 -> Switch1/1
  Stair Generator/1 -> Switch1/2, Switch2/2
  Switch1/1 -> MATLAB Function1/2(Q)
  Vref1 2/1 -> Switch2/1
  Pref/1 -> Switch2/3
  Switch2/1 -> MATLAB Function1/1(P)
  dq0 to abc/1 -> Gain1/1
  Gain1/1 -> Scope1/1
  connections:
  VSC (Average Model)/LConn3 -- L/LConn3
  L/RConn1 -- B1/LConn1
  Series RLC Branch1/RConn1 -- DC Voltage Source1/LConn1 -- Voltage Measurement1/LConn2 -- VSC (Average Model)/RConn2
  VSC (Average Model)/LConn1 -- L/LConn1
  L/RConn2 -- B1/LConn2
  VSC (Average Model)/LConn2 -- L/LConn2
  L/RConn3 -- B1/LConn3
  c/RConn1 -- B1/RConn3
  DC Voltage Source1/RConn1 -- Series RLC Branch1/LConn1 -- VSC (Average Model)/RConn1 -- Voltage Measurement1/LConn1
  B1/RConn1 -- a/RConn1
  B1/RConn2 -- b/RConn1

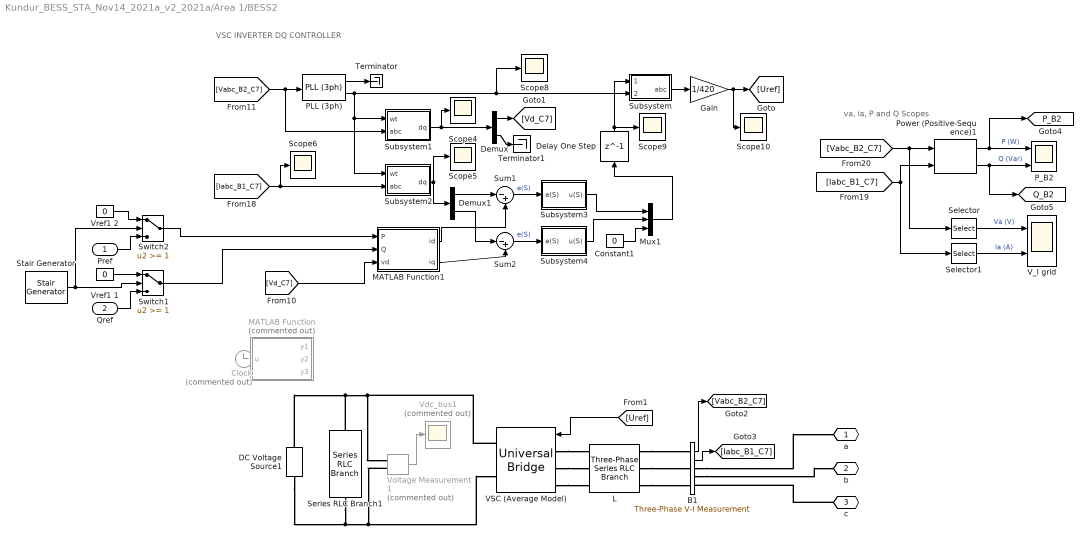
== system Kundur_BESS_STA_Nov14_2021a_v2_2021a/Area 1/BESS2  ==
  note: VSC INVERTER DQ CONTROLLER
  note: va, ia, P and Q Scopes
  Pref : Inport
  Qref : Inport  Port=2
  B1 : spsThreePhaseVIMeasurementLib/Three-Phase V-I Measurement  VoltageMeasurement=phase-to-ground  SetLabelV=off  LabelV=Vabc_B1  Vpu=off  VpuLL=off  CurrentMeasurement=yes  SetLabelI=off  LabelI=Iabc_B1_C7  Ipu=off  Pbase=100e6  Vbase=500e3  OutputType=Magnitude  PhasorSimulation=off  PSBequivalent=0
  Clock : Clock  Commented=on
  Constant1 : Constant  Value=0
  DC Voltage Source1 : spsDCVoltageSourceLib/DC Voltage Source  Amplitude=Vdc  Measurements=None
  Delay One Step : Delay  DelayLength=1
  Demux : Demux  Outputs=2
  Demux1 : Demux  Outputs=2
  Gain : Gain  Gain=1/420
  L : spsThreePhaseSeriesRLCBranchLib/Three-Phase Series RLC Branch  LConnTagsString=A|B|C  RConnTagsString=A|B|C  BranchType=RL  Resistance=500e-6*377/50/2  Inductance=1200e-6/2  Capacitance=inf  Measurements=None
  MATLAB Function : MATLAB Function  Commented=on  TreatAsAtomicUnit=on
  MATLAB Function1 : MATLAB Function  TreatAsAtomicUnit=on
  Mux1 : Mux  Inputs=3
  PLL (3ph) : spsPLL3phLib/PLL (3ph)  Fmin=58  Par_Init="[-0.57  60]"  ParK=[180, 3200, 1]  TcD=1e-4  MaxRateChangeFreq=12  FilterCutOffFreq=25  Ts=Ts  AGC=on
  P_B2 : Scope  NumInputPorts=2
  Power (Positive-Sequence)1 : spsPowerPositiveSequenceLib/Power (Positive-Sequence)  Freq=60  Vinit=[0, 0]  Iinit=[0, 0]  Ts=Ts
  Scope{4..6,8..10} (6 alike) : Scope
  Selector : Selector  InputPortWidth=3  IndexOptions=Index vector (dialog)  Indices=[1]  OutputSizes=1
  Selector1 : Selector  InputPortWidth=3  IndexOptions=Index vector (dialog)  Indices=[1]  OutputSizes=1
  Series RLC Branch1 : spsSeriesRLCBranchLib/Series RLC Branch  LConnTagsString=__new0  RConnTagsString=__new0  BranchType=RC  Resistance=1e-7  Inductance=1e-3  SetiL0=off  InitialCurrent=0  Capacitance=C  Setx0=off  InitialVoltage=400  Measurements=None
  Stair Generator : spsStairGeneratorLib/Stair Generator  t=[0 0.03]  e=[1 0]  Ts=0
  Subsystem : Subsystem
  Subsystem1 : Subsystem
  Subsystem2 : Subsystem
  Subsystem3 : Subsystem
  Subsystem4 : Subsystem
  Sum1 : Sum  Inputs=|-+
  Sum2 : Sum  Inputs=|-+
  Switch1 : Switch  Threshold=1  SaturateOnIntegerOverflow=off
  Switch2 : Switch  Threshold=1  SaturateOnIntegerOverflow=off
  Terminator : Terminator
  Terminator1 : Terminator
  VSC (Average Model) : spsUniversalBridgeLib/Universal Bridge  Arms=3  SnubberResistance=1e5  SnubberCapacitance=inf  Device=Average-model based VSC  Ron=1e-3  Lon=0  ForwardVoltages="[  0  0  ]"  ForwardVoltage=0  GTOparameters=[ 10e-6 , 20e-6 ]  IGBTparameters=[ 1e-6 , 2e-6 ]  Measurements=None  Measurements_2=None  converterType=Rectifier
  V_I grid : Scope  NumInputPorts=2
  Vdc_bus1 : Scope  Commented=on
  Voltage Measurement1 : spsVoltageMeasurementLib/Voltage Measurement  Commented=on  PhasorSimulation=off  OutputType=Complex  PSBequivalent=0
  Vref1 1 : Constant  Value=0
  Vref1 2 : Constant  Value=0
  a : PMIOPort  Side=Right
  b : PMIOPort  Port=2  Side=Right
  c : PMIOPort  Port=3  Side=Right
  tag scope: P_B2=global, Q_B2=global
  wires:
  Sum2/1 -> Subsystem4/1(e(S))  "e(S)"
  PLL (3ph)/2 -> Subsystem2/1(wt), Subsystem1/1(wt), Scope8/1, Subsystem/2(wt1)
  Voltage Measurement1/1 -> Vdc_bus1/1
  Mux1/1 -> Delay One Step/1
  Selector/1 -> V_I grid/1  "Va (V)"
  Delay One Step/1 -> Scope9/1, Subsystem/1(dq0)
  MATLAB Function1/1(id) -> Sum1/2
  Sum1/1 -> Subsystem3/1(e(S))  "e(S)"
  Subsystem4/1(u(S)) -> Mux1/2
  Power (Positive-Sequence)1/2 -> [Q_B2], P_B2/2  "Q (Var)"
  Demux/1 -> [Vd_C7]
  [Iabc_B1_C7] -> Scope6/1, Subsystem2/2(abc)
  Subsystem/1(abc) -> Gain/1
  [Vabc_B2_C7] -> Selector/1, Power (Positive-Sequence)1/1
  Subsystem3/1(u(S)) -> Mux1/1
  Gain/1 -> Scope10/1, [Uref]
  [Vabc_B2_C7] -> Subsystem1/2(abc), PLL (3ph)/1
  Selector1/1 -> V_I grid/2  "Ia (A)"
  Demux1/1 -> Sum1/1
  [Uref] -> VSC (Average Model)/1
  Demux/2 -> Terminator1/1
  [Iabc_B1_C7] -> Power (Positive-Sequence)1/2, Selector1/1
  Constant1/1 -> Mux1/3
  Subsystem1/1(dq) -> Demux/1, Scope4/1
  Demux1/2 -> Sum2/1
  Power (Positive-Sequence)1/1 -> [P_B2], P_B2/1  "P (W)"
  MATLAB Function1/2(iq) -> Sum2/2
  [Vd_C7] -> MATLAB Function1/3(vd)
  PLL (3ph)/1 -> Terminator/1
  Subsystem2/1(dq) -> Demux1/1, Scope5/1
  B1/1 -> [Vabc_B2_C7]
  B1/2 -> [Iabc_B1_C7]
  Clock/1 -> MATLAB Function/1(u)
  Qref/1 -> Switch1/3
  Vref1 1/1 -> Switch1/1
  Stair Generator/1 -> Switch1/2, Switch2/2
  Switch1/1 -> MATLAB Function1/2(Q)
  Vref1 2/1 -> Switch2/1
  Pref/1 -> Switch2/3
  Switch2/1 -> MATLAB Function1/1(P)
  connections:
  VSC (Average Model)/LConn3 -- L/LConn3
  L/RConn1 -- B1/LConn1
  Series RLC Branch1/RConn1 -- DC Voltage Source1/LConn1 -- Voltage Measurement1/LConn2 -- VSC (Average Model)/RConn2
  VSC (Average Model)/LConn1 -- L/LConn1
  L/RConn2 -- B1/LConn2
  VSC (Average Model)/LConn2 -- L/LConn2
  L/RConn3 -- B1/LConn3
  c/RConn1 -- B1/RConn3
  DC Voltage Source1/RConn1 -- Series RLC Branch1/LConn1 -- VSC (Average Model)/RConn1 -- Voltage Measurement1/LConn1
  B1/RConn1 -- a/RConn1
  B1/RConn2 -- b/RConn1
